simulink model "SimulacaoAula"  (R2014a)
settings: Solver=ode45  StartTime=0.0  StopTime=10  RelTol=1e-3
values from neighbouring files (symbols this model uses):
  KdT = 0    [init.m]
  KiT = 1 / 1    (= 1)    [init.m]
  KpT = 1 / ((1/4)*1)    (= 4)    [init.m]
libraries: cstblocks x2, simulink x1
settings Model: Creator=vpm-ssd  LastModifiedBy=vpm-ssd

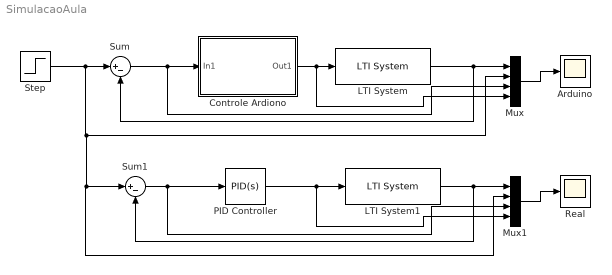
== system SimulacaoAula ==
  "Arduino " : Scope
  Controle Ardiono : Subsystem
  LTI System : cstblocks/LTI System  sys=pAulaTeorica  IC=[]
  LTI System1 : cstblocks/LTI System  sys=pAulaTeorica  IC=[]
  Mux : Mux
  Mux1 : Mux
  PID Controller : simulink/Continuous/PID Controller  Controller=PID  TimeDomain=Continuous-time  SampleTime=1  IntegratorMethod=Forward Euler  FilterMethod=Forward Euler  Form=Parallel  P=KpT  I=KpT/KiT  D=KdT  N=100  InitialConditionSource=internal  InitialConditionForIntegrator=0  InitialConditionForFilter=0  ExternalReset=none  LimitOutput=off  UpperSaturationLimit=inf  LowerSaturationLimit=-inf  LinearizeAsGain=on  AntiWindupMode=none  Kb=1  TrackingMode=off  Kt=1  PParamMin=[]  PParamMax=[]  IParamMin=[]  IParamMax=[]  DParamMin=[]  DParamMax=[]  NParamMin=[]  NParamMax=[]  KbParamMin=[]  KbParamMax=[]  KtParamMin=[]  KtParamMax=[]  POutMin=[]  POutMax=[]  IOutMin=[]  IOutMax=[]  DOutMin=[]  DOutMax=[]  NOutMin=[]  NOutMax=[]  KbOutMin=[]  KbOutMax=[]  KtOutMin=[]  KtOutMax=[]  IntegratorOutMin=[]  IntegratorOutMax=[]  FilterOutMin=[]  FilterOutMax=[]  SumOutMin=[]  SumOutMax=[]  SumI1OutMin=[]  SumI1OutMax=[]  SumI2OutMin=[]  SumI2OutMax=[]  SumI3OutMin=[]  SumI3OutMax=[]  SumDOutMin=[]  SumDOutMax=[]  SaturationOutMin=[]  SaturationOutMax=[]  IntegratorContinuousStateAttributes=''  IntegratorStateMustResolveToSignalObject=off  IntegratorRTWStateStorageClass=Auto  FilterContinuousStateAttributes=''  FilterStateMustResolveToSignalObject=off  FilterRTWStateStorageClass=Auto
  Real : Scope
  Step : Step  After=50  SampleTime=0
  Sum : Sum  Inputs=|+-
  Sum1 : Sum  Inputs=|+-
  wires:
  Sum/1 -> Mux/3, Controle Ardiono/1(In1)
  Controle Ardiono/1(Out1) -> Mux/4, LTI System/1
  Mux/1 -> "Arduino "/1
  LTI System/1 -> Sum/2, Mux/1
  Step/1 -> Mux1/2, Sum1/1, Mux/2, Sum/1
  Sum1/1 -> PID Controller/1, Mux1/3
  PID Controller/1 -> Mux1/4, LTI System1/1
  Mux1/1 -> Real/1
  LTI System1/1 -> Sum1/2, Mux1/1

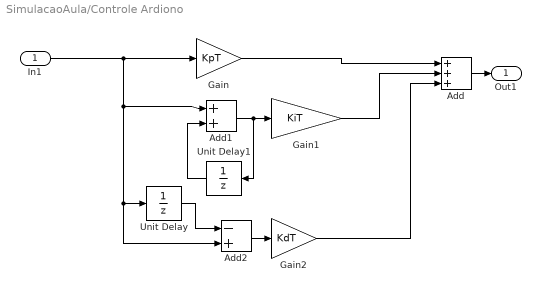
== system SimulacaoAula/Controle Ardiono ==
  In1 : Inport
  Add : Sum  Inputs=+++  SampleTime=0.1
  Add1 : Sum  SampleTime=0.1
  Add2 : Sum  Inputs=-+  SampleTime=0.1
  Gain : Gain  Gain=KpT  SampleTime=0.1
  Gain1 : Gain  Gain=KiT  SampleTime=0.1
  Gain2 : Gain  Gain=KdT  SampleTime=0.1
  Unit Delay : UnitDelay  SampleTime=0.1
  Unit Delay1 : UnitDelay  SampleTime=0.1
  Out1 : Outport
  wires:
  Gain2/1 -> Add/3
  Unit Delay/1 -> Add2/1
  Gain1/1 -> Add/2
  Add1/1 -> Unit Delay1/1, Gain1/1
  Add2/1 -> Gain2/1
  Add/1 -> Out1/1
  Gain/1 -> Add/1
  Unit Delay1/1 -> Add1/2
  In1/1 -> Add2/2, Unit Delay/1, Add1/1, Gain/1
